simulink model "ex4_statecart"  (R2024a)
settings: Solver=FixedStepDiscrete  StartTime=0.0  StopTime=10.0  FixedStep=0.1  RelTol=1e-3
settings Model: Creator=erfuu  LastModifiedBy=Mohammad Moein
settings SolverCC: AlgebraicLoopSolver=TrustRegion  AutoInsertRateTranBlk=on
settings DataIOCC: ExternalInput=sample_input.getElement('dec'),sample_input.getElement('inc'),sample_input.getElement('t_on'),sample_input.getElement('t_off'),sample_input.getElement('stop'),sample_input.getElement('start')  LimitDataPoints=on  LoadExternalInput=on
settings OptimizationCC: DefaultParameterBehavior=Inlined  EnhancedBackFolding=on  PassReuseOutputArgsAs=Individual arguments  ZeroExternalMemoryAtStartup=off  ZeroInternalMemoryAtStartup=off  MaxStackSize=64  OptimizeBlockOrder=speed  DifferentSizesBufferReuse=on  OptimizationCustomize=off  EfficientTunableParamExpr=on
settings DebuggingCC: ParameterTunabilityLossMsg=error  UnconnectedInputMsg=warning  UnconnectedOutputMsg=warning  UnconnectedLineMsg=warning  AllowSymbolicDim=off  SFUnexpectedBacktrackingDiag=warning  SFNoUnconditionalDefaultTransitionDiag=warning  SFExecutionAtInitializationDiag=none  UnderSpecifiedDimensionMsg=warning  ArithmeticOperatorsInVariantConditions=warning
settings HardwareCC: ProdBitPerInt=16  ProdBitPerPointer=16  ProdBitPerSizeT=16  ProdBitPerPtrDiffT=16  ProdLargestAtomicFloat=None  ProdWordSize=8  ProdHWDeviceType=Atmel->AVR
settings ModelReferenceCC: EnableRefExpFcnMdlSchedulingChecks=on
settings SFSimCC: SimUseLocalCustomCode=off  MATLABDynamicMemAlloc=off  CustomCodeUndefinedFunction=UseInterfaceOnly
settings RTWCC: Description=Embedded Coder  SystemTargetFile=ert.tlc  TemplateMakefile=ert_default_tmf  RTWUseLocalCustomCode=off  Toolchain=Arduino AVR  BuildConfiguration=Faster Runs  GPUComputeCapability=3.5  DLArmComputeVersion=19.05
settings CodeAppCC: ForceParamTrailComments=on  IgnoreCustomStorageClasses=off  OperatorAnnotations=on  SimulinkDataObjDesc=on  SFDataObjDesc=on  InsertBlockDesc=on
settings ERTTargetCC: SupportContinuousTime=on  ExtModeTransport=3  ExtModeStaticAlloc=on  ExtModeStaticAllocSize=2048  ExtModeMexFile=ext_xcp  ExtModeIntrfLevel=Level2 - Open  ERTCustomFileTemplate=example_file_process.tlc
settings ConfigComp: CovMetricSettings=dw  CovSaveCumulativeToWorkspaceVar=on  CovSaveSingleToWorkspaceVar=on  CovExternalEMLEnable=off  CovSFcnEnable=off

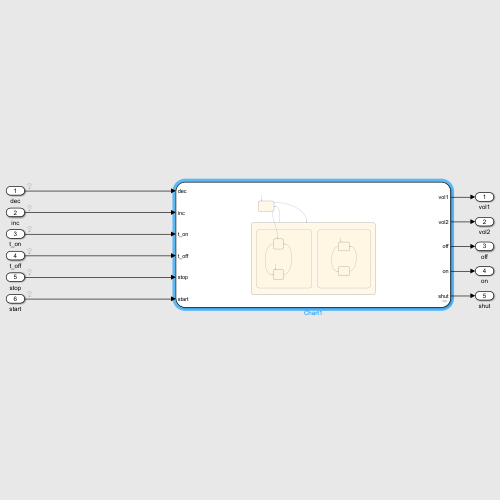
[thumbnail: Simulink's stored preview of the top-level diagram]
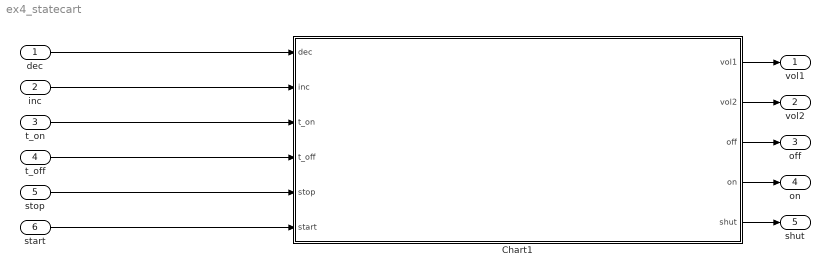
== system ex4_statecart ==
  dec : Inport
  inc : Inport  Port=2
  t_on : Inport  Port=3
  t_off : Inport  Port=4
  stop : Inport  Port=5
  start : Inport  Port=6
  Chart1 : Stateflow chart  TreatAsAtomicUnit=on
  vol1 : Outport
  vol2 : Outport  Port=2
  off : Outport  Port=3
  on : Outport  Port=4
  shut : Outport  Port=5
  wires:
  Chart1/1(vol1) -> vol1/1
  Chart1/2(vol2) -> vol2/1
  Chart1/3(off) -> off/1
  Chart1/4(on) -> on/1
  Chart1/5(shut) -> shut/1
  dec/1 -> Chart1/1(dec)
  inc/1 -> Chart1/2(inc)
  t_on/1 -> Chart1/3(t_on)
  t_off/1 -> Chart1/4(t_off)
  stop/1 -> Chart1/5(stop)
  start/1 -> Chart1/6(start)

== stateflow chart ex4_statecart/Chart1 ==
  state Shut
  state Op
    state Mode [parallel]
      settings: executionOrder=1
      state On
      state Off
      Off -> On : [t_on == 1]{off = 0; on = 1}
      On -> Off : [t_off == 1]{off = 1; on = 0}
      (default) -> Off : {off = 1; on = 0;}
    state Vol [parallel]
      settings: executionOrder=2
      state Vol1
      state Vol2
      (default) -> Vol1 : {vol1 = 1; vol2 = 0;}
      Vol2 -> Vol1 : [dec == 1]{vol1 = 1; vol2 = 0}
      Vol1 -> Vol2 : [inc == 1]{vol1 = 0; vol2 = 1}
  (default) -> Shut
  Shut -> Op [order 1] : [start == 1]{shut = 0;}
  Op -> Shut : [stop == 1]{shut = 1; vol1 = 0; vol2 = 0; on = 0; off=0;}
  Shut -> On [order 2] : [t_on == 1]{shut = 0; on = 1; off = 0;}
  data: dec input; inc input; t_on input; t_off input; stop input; start input; vol1 output =0; vol2 output =0; off output =0; on output =0; shut output =1
